simulink model "spherical_tank_controlled"  (R2017b)
settings: Solver=VariableStepAuto  StartTime=0.0  StopTime=200  RelTol=1e-3
values from neighbouring files (symbols this model uses):
  R = 900    [init_canonical.m]    (also in init_spherical.m = 30)
  Rr = 0.5    [init_spherical.m]
settings Model: Creator=Laci  LastModifiedBy=kn17063

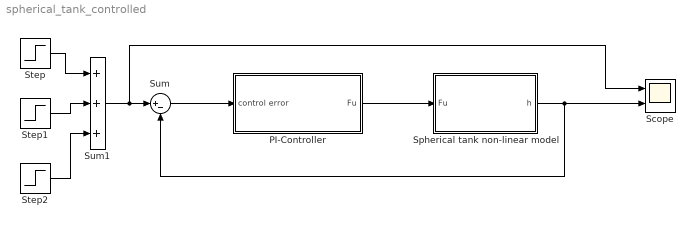
== system spherical_tank_controlled ==
  PI-Controller : Subsystem
  Scope : Scope  NumInputPorts=2
  Spherical tank non-linear model : Subsystem
  Step : Step  Time=10  Before=0.001  After=0.20  SampleTime=0
  Step1 : Step  Time=100  After=0.05  SampleTime=0
  Step2 : Step  Time=140  After=-0.05  SampleTime=0
  Sum : Sum  Inputs=|+-
  Sum1 : Sum  Inputs=+++
  wires:
  Spherical tank non-linear model/1(h) -> Scope/2, Sum/2
  Sum1/1 -> Scope/1, Sum/1
  Sum/1 -> PI-Controller/1(control error)
  PI-Controller/1(Fu) -> Spherical tank non-linear model/1(Fu)
  Step/1 -> Sum1/1
  Step1/1 -> Sum1/2
  Step2/1 -> Sum1/3

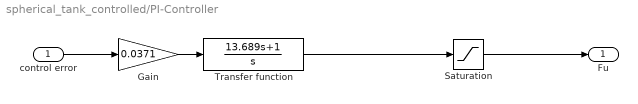
== system spherical_tank_controlled/PI-Controller ==
  control error : Inport
  Gain : Gain  Gain=0.0371
  Saturation : Saturate  UpperLimit=20e-3  LowerLimit=0
  Transfer function : TransferFcn  Numerator=[13.689 1]  Denominator=[1 0]
  Fu : Outport
  wires:
  control error/1 -> Gain/1
  Gain/1 -> Transfer function/1
  Transfer function/1 -> Saturation/1
  Saturation/1 -> Fu/1

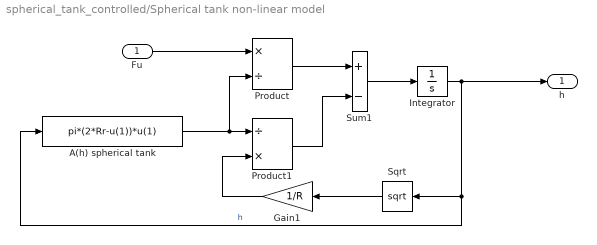
== system spherical_tank_controlled/Spherical tank non-linear model ==
  Fu : Inport
  A(h) spherical tank : Fcn  Expr=pi*(2*Rr-u(1))*u(1)
  Gain1 : Gain  Gain=1/R
  Integrator : Integrator  InitialCondition=1e-3
  Product : Product  Inputs=*/
  Product1 : Product  Inputs=/*
  Sqrt : Sqrt  SaturateOnIntegerOverflow=on
  Sum1 : Sum  Inputs=+-
  h : Outport
  wires:
  Gain1/1 -> Product1/2
  Fu/1 -> Product/1
  A(h) spherical tank/1 -> Product/2, Product1/1
  Sqrt/1 -> Gain1/1
  Sum1/1 -> Integrator/1
  Product1/1 -> Sum1/2
  Product/1 -> Sum1/1
  Integrator/1 -> h/1, A(h) spherical tank/1, Sqrt/1  "h"
